simulink model "M01_HPP_Control"  (R2017b)
settings: Solver=FixedStepAuto  StartTime=0.0  StopTime=10.0  RelTol=1e-3
libraries: simulink x4
settings Model: Creator=Пользователь  LastModifiedBy=pavel.dushkin
settings OptimizationCC: DefaultParameterBehavior=Inlined  UseDivisionForNetSlopeComputation=on  UseFloatMulNetSlope=on  InlineInvariantSignals=on  PassReuseOutputArgsAs=Individual arguments  ZeroExternalMemoryAtStartup=off  ZeroInternalMemoryAtStartup=off  NoFixptDivByZeroProtection=on  EfficientFloat2IntCast=on  LifeSpan=1
settings DebuggingCC: ParameterTunabilityLossMsg=error
settings HardwareCC: ProdBitPerPointer=32  ProdBitPerSizeT=32  ProdBitPerPtrDiffT=32  ProdLargestAtomicInteger=Long  ProdLargestAtomicFloat=Double  ProdWordSize=32  ProdLongLongMode=on  ProdHWDeviceType=ARM Compatible->ARM Cortex
settings SFSimCC: MATLABDynamicMemAlloc=off
settings RTWCC: SystemTargetFile=ert.tlc  GenCodeOnly=on  TemplateMakefile=ert_default_tmf  IncludeHyperlinkInReport=on
settings CodeAppCC: IgnoreCustomStorageClasses=off  MaxIdLength=127  SimulinkDataObjDesc=on  SFDataObjDesc=on  MATLABFcnDesc=on  CustomSymbolStrGlobalVar=rt$N$M  CustomSymbolStrType=$N$M  CustomSymbolStrFcn=$N$M$F  CustomSymbolStrMacro=$N$M  InsertBlockDesc=on  StateflowObjectComments=on
settings ERTTargetCC: TargetLangStandard=C99 (ISO)  IncludeMdlTerminateFcn=off  CombineSignalStateStructs=on  SuppressErrorStatus=on  SupportNonInlinedSFcns=on  InlinedParameterPlacement=NonHierarchical  ERTCustomFileTemplate=example_file_process.tlc  ERTFilePackagingFormat=Compact  PreserveExpressionOrder=on  PreserveIfCondition=on  SuppressUnreachableDefaultCases=off  MemSecPackage=Simulink  MemSecDataConstants=MemVolatile

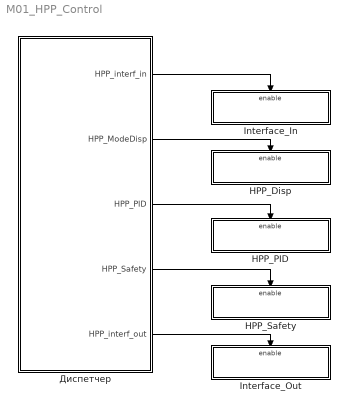
== system M01_HPP_Control ==
  HPP_Disp : Subsystem
  HPP_PID : Subsystem
  HPP_Safety : Subsystem
  Interface_In : Subsystem
  Interface_Out : Subsystem
  Диспетчер : Stateflow chart  TreatAsAtomicUnit=on
  wires:
  Диспетчер/3(HPP_PID) -> HPP_PID/Enable
  Диспетчер/2(HPP_ModeDisp) -> HPP_Disp/Enable
  Диспетчер/4(HPP_Safety) -> HPP_Safety/Enable
  Диспетчер/1(HPP_interf_in) -> Interface_In/Enable
  Диспетчер/5(HPP_interf_out) -> Interface_Out/Enable

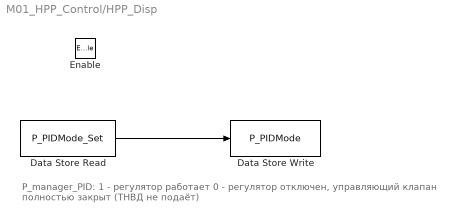
== system M01_HPP_Control/HPP_Disp ==
  note: P_manager_PID:
      | 1 - регулятор работает
      | 0 - регулятор отключен, управляющий клапан полностью закрыт (ТНВД не подаёт)
  Enable : EnablePort
  Data Store Read : DataStoreRead  DataStoreName=P_PIDMode_Set
  Data Store Write : DataStoreWrite  DataStoreName=P_PIDMode
  wires:
  Data Store Read/1 -> Data Store Write/1

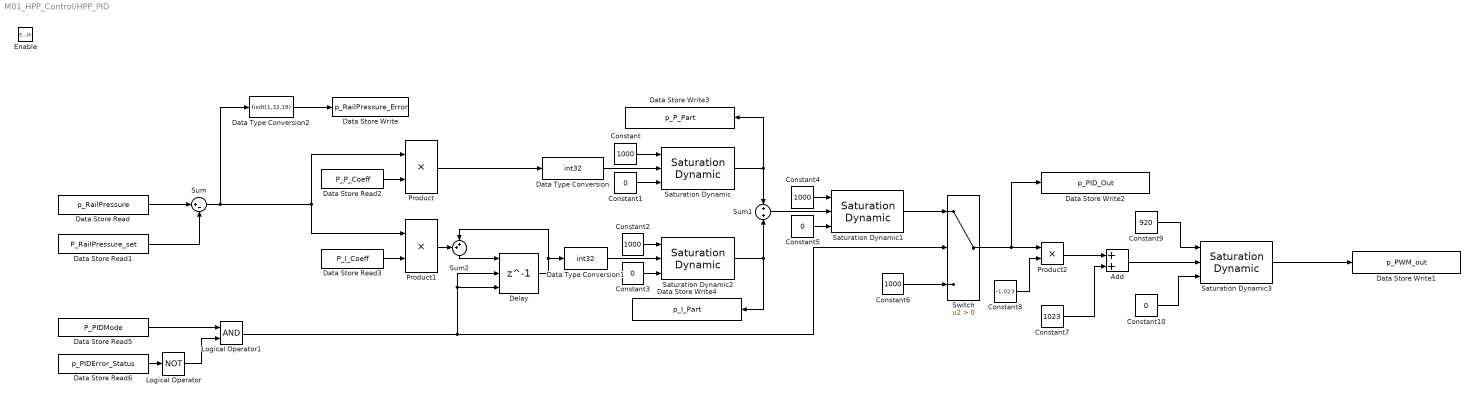
== system M01_HPP_Control/HPP_PID ==
  Enable : EnablePort
  Add : Sum  OutDataTypeStr=int32
  Constant{,2,4,6} (4 alike) : Constant  Value=1000  OutDataTypeStr=int32
  Constant{1,3,5,10} (4 alike) : Constant  Value=0  OutDataTypeStr=int32
  Constant7 : Constant  Value=1023  OutDataTypeStr=int32
  Constant8 : Constant  Value=-1.023  OutDataTypeStr=fixdt(1,32,18)
  Constant9 : Constant  Value=920  OutDataTypeStr=int32
  Data Store Read : DataStoreRead  DataStoreName=p_RailPressure
  Data Store Read1 : DataStoreRead  DataStoreName=P_RailPressure_set  DataStoreElements=P_RailPressure_set
  Data Store Read2 : DataStoreRead  DataStoreName=P_P_Coeff
  Data Store Read3 : DataStoreRead  DataStoreName=P_I_Coeff
  Data Store Read5 : DataStoreRead  DataStoreName=P_PIDMode
  Data Store Read6 : DataStoreRead  DataStoreName=p_PIDError_Status
  Data Store Write : DataStoreWrite  DataStoreName=p_RailPressure_Error
  Data Store Write1 : DataStoreWrite  DataStoreName=p_PWM_out
  Data Store Write2 : DataStoreWrite  DataStoreName=p_PID_Out
  Data Store Write3 : DataStoreWrite  DataStoreName=p_P_Part
  Data Store Write4 : DataStoreWrite  DataStoreName=p_I_Part
  Data Type Conversion : DataTypeConversion  OutDataTypeStr=int32
  Data Type Conversion1 : DataTypeConversion  OutDataTypeStr=int32
  Data Type Conversion2 : DataTypeConversion  OutDataTypeStr=fixdt(1,32,18)
  Delay : Delay  DelayLength=1  InitialCondition=0  ExternalReset=Falling  ShowEnablePort=on  InputProcessing=Inherited
      settings: InputPortMap=u0,e6,r5
  Logical Operator : Logic  Operator=NOT  AllPortsSameDT=off  OutDataTypeStr=boolean
  Logical Operator1 : Logic  AllPortsSameDT=off  OutDataTypeStr=boolean
  Product : Product  OutDataTypeStr=Inherit: Same as first input
  Product1 : Product  OutDataTypeStr=Inherit: Same as first input
  Product2 : Product  OutDataTypeStr=fixdt(0,32,18)
  Saturation Dynamic{,1..3} (4 alike) : simulink/Discontinuities/Saturation Dynamic  OutMin=[]  OutMax=[]  OutDataTypeStr=Inherit: Same as second input  OutDataType=fixdt(1, 16)  OutScaling=2^-10  DoSatur=off
  Sum : Sum  Inputs=|+-  OutDataTypeStr=Inherit: Same as first input
  Sum1 : Sum  OutDataTypeStr=int32
  Sum2 : Sum  Inputs=++|
  Switch : Switch  Criteria=u2 > Threshold
  wires:
  Saturation Dynamic1/1 -> Switch/1
  Sum1/1 -> Saturation Dynamic1/2
  Data Store Read3/1 -> Product1/2
  Constant6/1 -> Switch/3
  Saturation Dynamic2/1 -> Sum1/2, Data Store Write4/1
  Sum/1 -> Data Type Conversion2/1, Product1/1, Product/1
  Data Store Read2/1 -> Product/2
  Data Store Read/1 -> Sum/1
  Constant3/1 -> Saturation Dynamic2/3
  Saturation Dynamic/1 -> Data Store Write3/1, Sum1/1
  Logical Operator1/1 -> Switch/2, Delay/3, Delay/2
  Constant4/1 -> Saturation Dynamic1/1
  Data Store Read1/1 -> Sum/2
  Product1/1 -> Sum2/1
  Constant2/1 -> Saturation Dynamic2/1
  Constant1/1 -> Saturation Dynamic/3
  Product/1 -> Data Type Conversion/1
  Constant5/1 -> Saturation Dynamic1/3
  Sum2/1 -> Delay/1
  Constant/1 -> Saturation Dynamic/1
  Delay/1 -> Sum2/2, Data Type Conversion1/1
  Data Store Read5/1 -> Logical Operator1/1
  Logical Operator/1 -> Logical Operator1/2
  Data Store Read6/1 -> Logical Operator/1
  Switch/1 -> Product2/1, Data Store Write2/1
  Constant8/1 -> Product2/2
  Product2/1 -> Add/1
  Constant7/1 -> Add/2
  Add/1 -> Saturation Dynamic3/2
  Saturation Dynamic3/1 -> Data Store Write1/1
  Constant9/1 -> Saturation Dynamic3/1
  Constant10/1 -> Saturation Dynamic3/3
  Data Type Conversion/1 -> Saturation Dynamic/2
  Data Type Conversion1/1 -> Saturation Dynamic2/2
  Data Type Conversion2/1 -> Data Store Write/1

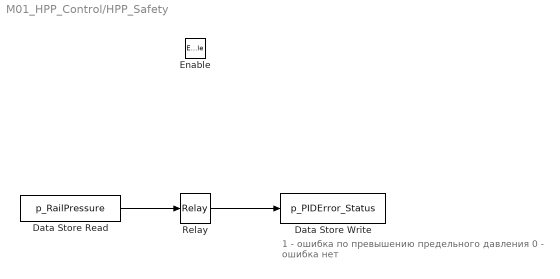
== system M01_HPP_Control/HPP_Safety ==
  note: 1 - ошибка по превышению предельного давления
      | 0 - ошибка нет
  Enable : EnablePort
  Data Store Read : DataStoreRead  DataStoreName=p_RailPressure
  Data Store Write : DataStoreWrite  DataStoreName=p_PIDError_Status
  Relay : Relay  OnSwitchValue=1700  OffSwitchValue=1500  OutDataTypeStr=boolean
  wires:
  Data Store Read/1 -> Relay/1
  Relay/1 -> Data Store Write/1

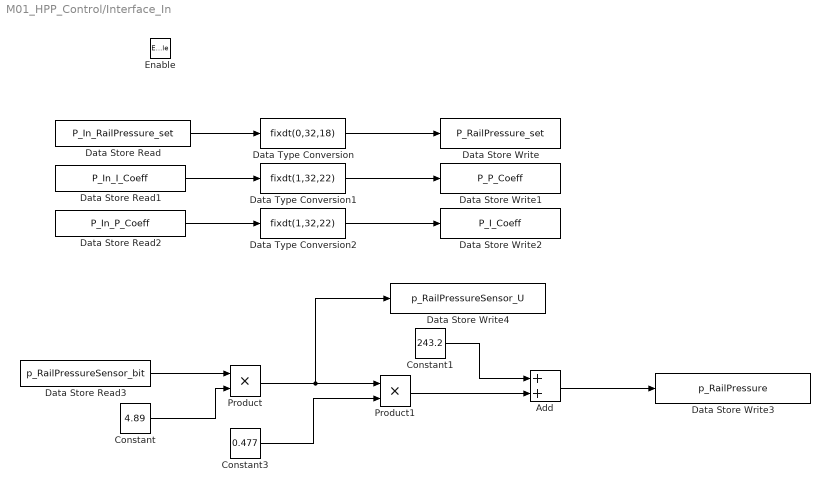
== system M01_HPP_Control/Interface_In ==
  Enable : EnablePort
  Add : Sum  OutDataTypeStr=Inherit: Same as first input
  Constant : Constant  Value=4.89  OutDataTypeStr=fixdt(0,32,18)
  Constant1 : Constant  Value=243.2  OutDataTypeStr=fixdt(0,32,18)
  Constant3 : Constant  Value=0.477  OutDataTypeStr=fixdt(0,32,18)
  Data Store Read : DataStoreRead  DataStoreName=P_In_RailPressure_set
  Data Store Read1 : DataStoreRead  DataStoreName=P_In_I_Coeff
  Data Store Read2 : DataStoreRead  DataStoreName=P_In_P_Coeff
  Data Store Read3 : DataStoreRead  DataStoreName=p_RailPressureSensor_bit
  Data Store Write : DataStoreWrite  DataStoreName=P_RailPressure_set
  Data Store Write1 : DataStoreWrite  DataStoreName=P_P_Coeff
  Data Store Write2 : DataStoreWrite  DataStoreName=P_I_Coeff
  Data Store Write3 : DataStoreWrite  DataStoreName=p_RailPressure
  Data Store Write4 : DataStoreWrite  DataStoreName=p_RailPressureSensor_U
  Data Type Conversion : DataTypeConversion  OutDataTypeStr=fixdt(0,32,18)
  Data Type Conversion1 : DataTypeConversion  OutDataTypeStr=fixdt(1,32,22)
  Data Type Conversion2 : DataTypeConversion  OutDataTypeStr=fixdt(1,32,22)
  Product : Product  OutDataTypeStr=Inherit: Same as first input
  Product1 : Product  OutDataTypeStr=Inherit: Same as first input
  wires:
  Data Store Read/1 -> Data Type Conversion/1
  Data Type Conversion/1 -> Data Store Write/1
  Data Store Read1/1 -> Data Type Conversion1/1
  Data Store Read2/1 -> Data Type Conversion2/1
  Data Type Conversion2/1 -> Data Store Write2/1
  Data Type Conversion1/1 -> Data Store Write1/1
  Data Store Read3/1 -> Product/1
  Constant/1 -> Product/2
  Constant3/1 -> Product1/2
  Constant1/1 -> Add/1
  Product1/1 -> Add/2
  Product/1 -> Data Store Write4/1, Product1/1
  Add/1 -> Data Store Write3/1

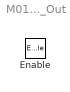
== system M01_HPP_Control/Interface_Out ==
  Enable : EnablePort

== stateflow chart M01_HPP_Control/Диспетчер ==
  (junction 123) -> (junction 124) : {
      | HPP_interf_in;
      | HPP_ModeDisp;
      | HPP_PID;
      | HPP_Safety;
      | HPP_interf_out;
      | }
  events: HPP_interf_in output EITHER_EDGE_EVENT; HPP_ModeDisp output EITHER_EDGE_EVENT; HPP_PID output EITHER_EDGE_EVENT; HPP_Safety output EITHER_EDGE_EVENT; HPP_interf_out output EITHER_EDGE_EVENT
